simulink model "task2"  (R2018b)
settings: Solver=VariableStepAuto  StartTime=0.0  StopTime=10.0  FixedStep=0.01  RelTol=1e-3
values from neighbouring files (symbols this model uses):
  F_c = 1.5    [task2.m]
  F_s = 1.75    [task2.m]
  F_v = 0.1    [task2.m]
  m = 2    [task2.m]
  sigma_0 = 750    [task2.m]
  sigma_1 = 10    [task2.m]
  sigma_2 = F_v    (= 0.1)    [task2.m]
  v_s = 0.2    [task2.m]
libraries: simulink x5
settings Model: Creator=Torbjorn  LastModifiedBy=Torbjorn

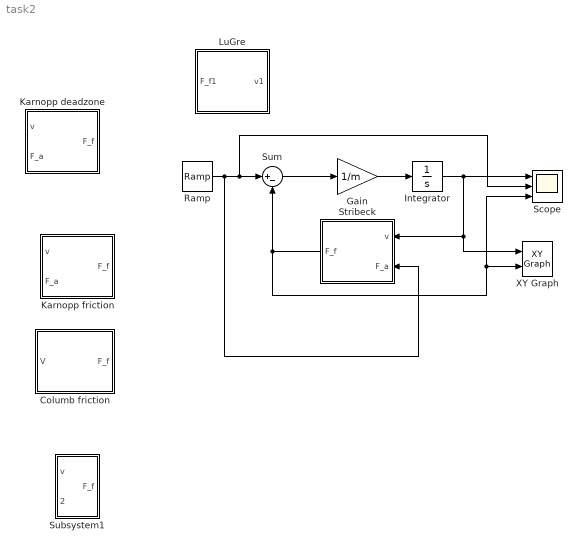
== system task2 ==
  Columb friction : Subsystem
  Gain : Gain  Gain=1/m
  Integrator : Integrator
  Karnopp deadzone : Subsystem
  Karnopp friction : Subsystem
  LuGre : Subsystem
  Ramp : simulink/Sources/Ramp  slope=1  start=0  InitialOutput=0
  Scope : Scope  NumInputPorts=3
  Stribeck : Subsystem
  Subsystem1 : Subsystem
  Sum : Sum  Inputs=|+-
  XY Graph : simulink/Sinks/XY Graph  xmin=-1  xmax=1  ymin=-1  ymax=1  st=-1
  wires:
  Sum/1 -> Gain/1
  Gain/1 -> Integrator/1
  Integrator/1 -> XY Graph/1, Stribeck/1(v), Scope/1
  Ramp/1 -> Stribeck/2(F_a), Scope/2, Sum/1
  Stribeck/1(F_f) -> Scope/3, XY Graph/2, Sum/2

== system task2/Columb friction ==
  V : Inport
  Gain1 : Gain  Gain=F_c
  Sign : Signum
  F_f : Outport
  wires:
  Gain1/1 -> F_f/1
  V/1 -> Sign/1
  Sign/1 -> Gain1/1

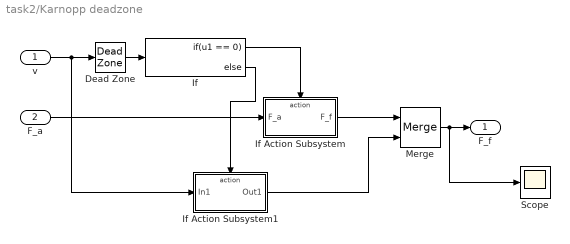
== system task2/Karnopp deadzone ==
  v : Inport
  F_a : Inport  Port=2
  Dead Zone : DeadZone  LowerValue=-1  UpperValue=1  SaturateOnIntegerOverflow=on
  If : If  IfExpression=u1 == 0  ZeroCross=off
  If Action Subsystem : Subsystem  TreatAsAtomicUnit=on
  If Action Subsystem1 : Subsystem  TreatAsAtomicUnit=on
  Merge : Merge
  Scope : Scope
  F_f : Outport
  wires:
  v/1 -> Dead Zone/1, If Action Subsystem1/1(In1)
  If/1 -> If Action Subsystem/Action
  F_a/1 -> If Action Subsystem/1(F_a)
  If Action Subsystem/1(F_f) -> Merge/1
  Merge/1 -> Scope/1, F_f/1
  If/2 -> If Action Subsystem1/Action
  If Action Subsystem1/1(Out1) -> Merge/2
  Dead Zone/1 -> If/1

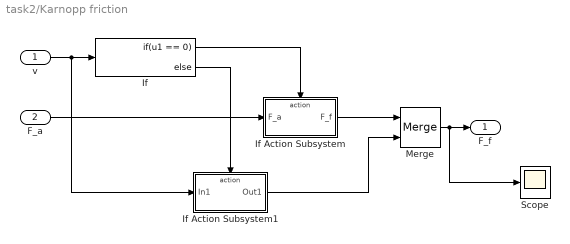
== system task2/Karnopp friction ==
  v : Inport
  F_a : Inport  Port=2
  If : If  IfExpression=u1 == 0
  If Action Subsystem : Subsystem  TreatAsAtomicUnit=on
  If Action Subsystem1 : Subsystem  TreatAsAtomicUnit=on
  Merge : Merge
  Scope : Scope
  F_f : Outport
  wires:
  v/1 -> If Action Subsystem1/1(In1), If/1
  If/1 -> If Action Subsystem/Action
  F_a/1 -> If Action Subsystem/1(F_a)
  If Action Subsystem/1(F_f) -> Merge/1
  Merge/1 -> Scope/1, F_f/1
  If/2 -> If Action Subsystem1/Action
  If Action Subsystem1/1(Out1) -> Merge/2

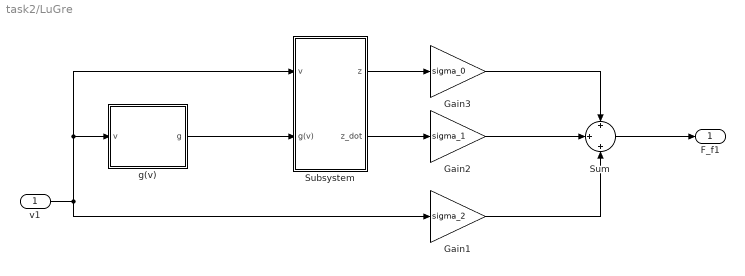
== system task2/LuGre ==
  v1 : Inport
  Gain1 : Gain  Gain=sigma_2
  Gain2 : Gain  Gain=sigma_1
  Gain3 : Gain  Gain=sigma_0
  Subsystem : Subsystem
  Sum : Sum  Inputs=+|+|+
  g(v) : Subsystem
  F_f1 : Outport
  wires:
  v1/1 -> g(v)/1(v), Subsystem/1(v), Gain1/1
  Gain2/1 -> Sum/2
  Subsystem/1(z) -> Gain3/1
  Sum/1 -> F_f1/1
  Subsystem/2(z_dot) -> Gain2/1
  Gain1/1 -> Sum/3
  g(v)/1(g) -> Subsystem/2(g(v))
  Gain3/1 -> Sum/1

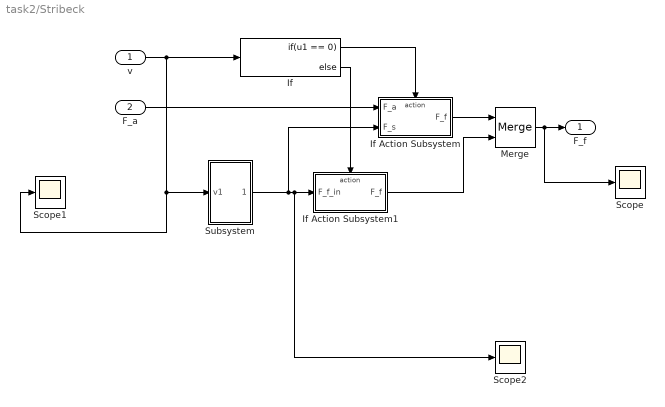
== system task2/Stribeck ==
  v : Inport
  F_a : Inport  Port=2
  If : If  IfExpression=u1 == 0
  If Action Subsystem : Subsystem  TreatAsAtomicUnit=on
  If Action Subsystem1 : Subsystem  TreatAsAtomicUnit=on
  Merge : Merge
  Scope : Scope
  Scope1 : Scope
  Scope2 : Scope
  Subsystem : Subsystem
  F_f : Outport
  wires:
  If/1 -> If Action Subsystem/Action
  F_a/1 -> If Action Subsystem/1(F_a)
  If Action Subsystem/1(F_f) -> Merge/1
  Merge/1 -> Scope/1, F_f/1
  If/2 -> If Action Subsystem1/Action
  If Action Subsystem1/1(F_f) -> Merge/2
  v/1 -> If/1, Subsystem/1(v1), Scope1/1
  Subsystem/1(F_f1) -> If Action Subsystem/2("F_s "), Scope2/1, If Action Subsystem1/1(F_f_in)

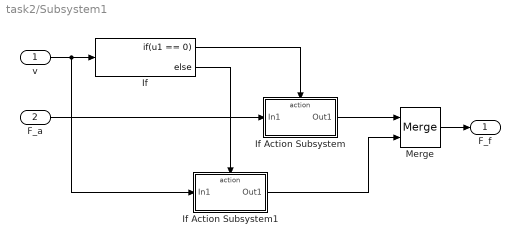
== system task2/Subsystem1 ==
  v : Inport
  F_a : Inport  Port=2
  If : If  IfExpression=u1 == 0
  If Action Subsystem : Subsystem  TreatAsAtomicUnit=on
  If Action Subsystem1 : Subsystem  TreatAsAtomicUnit=on
  Merge : Merge
  F_f : Outport
  wires:
  v/1 -> If Action Subsystem1/1(In1), If/1
  If/1 -> If Action Subsystem/Action
  F_a/1 -> If Action Subsystem/1(In1)
  If Action Subsystem/1(Out1) -> Merge/1
  Merge/1 -> F_f/1
  If/2 -> If Action Subsystem1/Action
  If Action Subsystem1/1(Out1) -> Merge/2

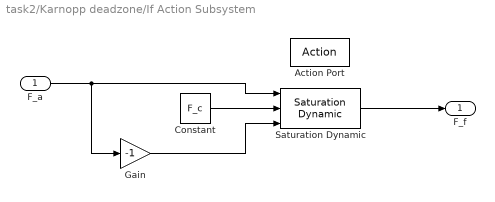
== system task2/Karnopp deadzone/If Action Subsystem ==
  F_a : Inport
  Action Port : ActionPort  ActionType=then
  Constant : Constant  Value=F_c
  Gain : Gain  Gain=-1
  Saturation Dynamic : simulink/Discontinuities/Saturation Dynamic  OutMin=[]  OutMax=[]  OutDataTypeStr=Inherit: Same as second input  OutDataType=fixdt(1, 16)  OutScaling=2^-10  DoSatur=off
  F_f : Outport
  wires:
  F_a/1 -> Gain/1, Saturation Dynamic/1
  Constant/1 -> Saturation Dynamic/2
  Gain/1 -> Saturation Dynamic/3
  Saturation Dynamic/1 -> F_f/1

== system task2/Karnopp deadzone/If Action Subsystem1 ==
  In1 : Inport
  Action Port : ActionPort  ActionType=else
  "Columb friction " : Subsystem
  Out1 : Outport
  wires:
  "Columb friction "/1(F_f) -> Out1/1
  In1/1 -> "Columb friction "/1(V)

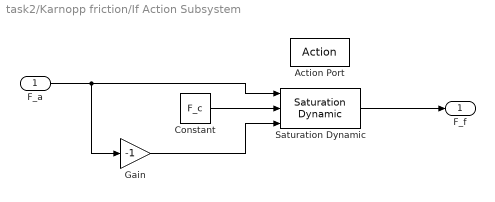
== system task2/Karnopp friction/If Action Subsystem ==
  F_a : Inport
  Action Port : ActionPort  ActionType=then
  Constant : Constant  Value=F_c
  Gain : Gain  Gain=-1
  Saturation Dynamic : simulink/Discontinuities/Saturation Dynamic  OutMin=[]  OutMax=[]  OutDataTypeStr=Inherit: Same as second input  OutDataType=fixdt(1, 16)  OutScaling=2^-10  DoSatur=off
  F_f : Outport
  wires:
  F_a/1 -> Gain/1, Saturation Dynamic/1
  Constant/1 -> Saturation Dynamic/2
  Gain/1 -> Saturation Dynamic/3
  Saturation Dynamic/1 -> F_f/1

== system task2/Karnopp friction/If Action Subsystem1 ==
  In1 : Inport
  Action Port : ActionPort  ActionType=else
  "Columb friction " : Subsystem
  Out1 : Outport
  wires:
  "Columb friction "/1(F_f) -> Out1/1
  In1/1 -> "Columb friction "/1(V)

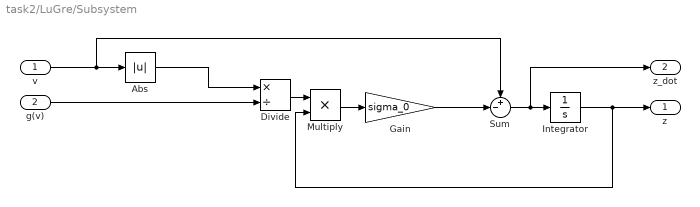
== system task2/LuGre/Subsystem ==
  v : Inport
  g(v) : Inport  Port=2
  Abs : Abs
  Divide : Product  Inputs=*/
  Gain : Gain  Gain=sigma_0
  Integrator : Integrator
  Multiply : Product
  Sum : Sum  Inputs=+-|
  z : Outport
  z_dot : Outport  Port=2
  wires:
  g(v)/1 -> Divide/2
  v/1 -> Sum/1, Abs/1
  Abs/1 -> Divide/1
  Divide/1 -> Multiply/1
  Multiply/1 -> Gain/1
  Gain/1 -> Sum/2
  Integrator/1 -> Multiply/2, z/1
  Sum/1 -> z_dot/1, Integrator/1

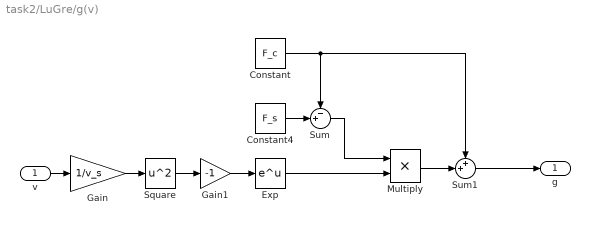
== system task2/LuGre/g(v) ==
  v : Inport
  Constant : Constant  Value=F_c
  Constant4 : Constant  Value=F_s
  Exp : Math  SaturateOnIntegerOverflow=on
  Gain : Gain  Gain=1/v_s
  Gain1 : Gain  Gain=-1
  Multiply : Product
  Square : Math  Operator=square  SaturateOnIntegerOverflow=on
  Sum : Sum  Inputs=-+|
  Sum1 : Sum  Inputs=++|
  g : Outport
  wires:
  v/1 -> Gain/1
  Gain1/1 -> Exp/1
  Sum/1 -> Multiply/1
  Exp/1 -> Multiply/2
  Constant4/1 -> Sum/2
  Gain/1 -> Square/1
  Square/1 -> Gain1/1
  Multiply/1 -> Sum1/2
  Sum1/1 -> g/1
  Constant/1 -> Sum/1, Sum1/1

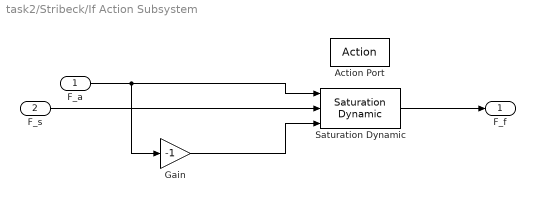
== system task2/Stribeck/If Action Subsystem ==
  F_a : Inport
  "F_s " : Inport  Port=2
  Action Port : ActionPort  ActionType=then
  Gain : Gain  Gain=-1
  Saturation Dynamic : simulink/Discontinuities/Saturation Dynamic  OutMin=[]  OutMax=[]  OutDataTypeStr=Inherit: Same as second input  OutDataType=fixdt(1, 16)  OutScaling=2^-10  DoSatur=off
  F_f : Outport
  wires:
  F_a/1 -> Gain/1, Saturation Dynamic/1
  "F_s "/1 -> Saturation Dynamic/2
  Gain/1 -> Saturation Dynamic/3
  Saturation Dynamic/1 -> F_f/1

== system task2/Stribeck/If Action Subsystem1 ==
  F_f_in : Inport
  Action Port : ActionPort  ActionType=else
  F_f : Outport
  wires:
  F_f_in/1 -> F_f/1

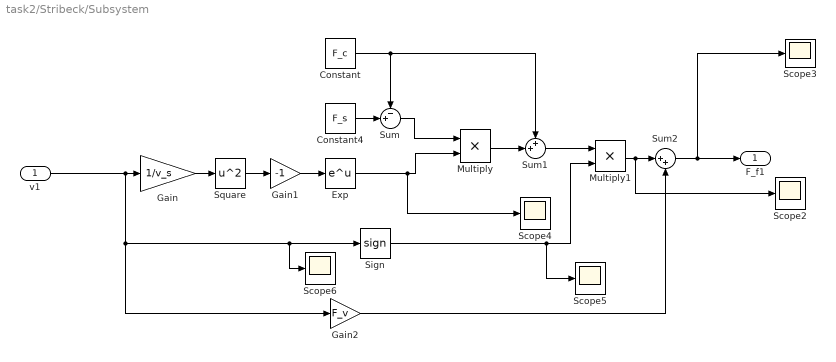
== system task2/Stribeck/Subsystem ==
  v1 : Inport
  Constant : Constant  Value=F_c
  Constant4 : Constant  Value=F_s
  Exp : Math  SaturateOnIntegerOverflow=on
  Gain : Gain  Gain=1/v_s
  Gain1 : Gain  Gain=-1
  Gain2 : Gain  Gain=F_v
  Multiply : Product
  Multiply1 : Product
  Scope{2..6} (5 alike) : Scope
  Sign : Signum  ZeroCross=off
  Square : Math  Operator=square  SaturateOnIntegerOverflow=on
  Sum : Sum  Inputs=-+|
  Sum1 : Sum  Inputs=++|
  Sum2 : Sum  Inputs=|++
  F_f1 : Outport
  wires:
  Gain/1 -> Square/1
  Sum1/1 -> Multiply1/1
  Sum2/1 -> F_f1/1, Scope3/1
  Gain1/1 -> Exp/1
  Constant4/1 -> Sum/2
  Gain2/1 -> Sum2/2
  Constant/1 -> Sum/1, Sum1/1
  Sum/1 -> Multiply/1
  Exp/1 -> Scope4/1, Multiply/2
  Multiply/1 -> Sum1/2
  Sign/1 -> Scope5/1, Multiply1/2
  Multiply1/1 -> Scope2/1, Sum2/1
  v1/1 -> Gain2/1, Scope6/1, Sign/1, Gain/1
  Square/1 -> Gain1/1

== system task2/Subsystem1/If Action Subsystem ==
  In1 : Inport
  Action Port : ActionPort  ActionType=then
  Saturation : Saturate  UpperLimit=F_c  LowerLimit=F_c
  Out1 : Outport
  wires:
  In1/1 -> Saturation/1
  Saturation/1 -> Out1/1

== system task2/Subsystem1/If Action Subsystem1 ==
  In1 : Inport
  Action Port : ActionPort  ActionType=else
  "Columb friction " : Subsystem
  Out1 : Outport
  wires:
  "Columb friction "/1(F_f) -> Out1/1
  In1/1 -> "Columb friction "/1(V)

== system task2/Karnopp deadzone/If Action Subsystem1/Columb friction  ==
  V : Inport
  Gain1 : Gain  Gain=F_c
  Sign : Signum  ZeroCross=off
  F_f : Outport
  wires:
  Gain1/1 -> F_f/1
  V/1 -> Sign/1
  Sign/1 -> Gain1/1

== system task2/Karnopp friction/If Action Subsystem1/Columb friction  ==
  V : Inport
  Gain1 : Gain  Gain=F_c
  Sign : Signum
  F_f : Outport
  wires:
  Gain1/1 -> F_f/1
  V/1 -> Sign/1
  Sign/1 -> Gain1/1

== system task2/Subsystem1/If Action Subsystem1/Columb friction  ==
  V : Inport
  Gain1 : Gain  Gain=F_c
  Sign : Signum
  F_f : Outport
  wires:
  Gain1/1 -> F_f/1
  V/1 -> Sign/1
  Sign/1 -> Gain1/1
